simulink model "Model"  (R2023b)
settings: Solver=ode4  StartTime=0.0  StopTime=100  FixedStep=0.01  RelTol=1e-3
values from neighbouring files (symbols this model uses):
  D = sqrt(px*px + py*py)    [test2.m]
undefined symbols (not defined in the file or in its folder): X, Y, Z
libraries: nesl_utility x41, sm_lib x34, simulink_extras x10, sharedtransform x1
(part 2 of 2)

== matlab function Model/MATLAB Function1 ==
  data: theta input; J output
function J = jacobian_3link(theta)
    L0 = 0.04494;
    L1 = 0.08979;
    L2 = 0.1665;
    L3a = 0.02945;
    L3b = 0.1232;

    t0 = theta(1);
    t1 = theta(2);
    t2 = theta(3);
    t01 = t0 + t1;
    t012 = t01 + t2;

    Rp = @(theta) [-sin(theta); cos(theta)]; 

    J1 =  L0 * Rp(t0 + pi/2) ...
         +L1 * Rp(t0) ...
         +L2 * Rp(t01) ...
         +L3a * Rp(t012 + pi/2) ...
         +L3b * Rp(t012);

    J2 =  L2 * Rp(t01) ...
         +L3a * Rp(t012 + pi/2) ...
         +L3b * Rp(t012);

    J3 =  L3a * Rp(t012 + pi/2) ...
         +L3b * Rp(t012);

    J = [J1, J2, J3];
end

== matlab function Model/MATLAB Function ==
  data: theta input; pos output
function pos = fk_3link_explicit(theta)
    L0 = 0.04494;
    L1 = 0.08979;
    L2 = 0.1665;
    L3a = 0.02945;
    L3b = 0.1232;

    t0 = theta(1);
    t1 = theta(2);
    t2 = theta(3);
    t01 = t0 + t1;
    t012 = t01 + t2;

    R = @(theta) [cos(theta); sin(theta)];

    P0 = [0; 0];
    P1 = P0 + L0 * R(t0 + pi/2);
    P2 = P1 + L1 * R(t0);
    P3 = P2 + L2 * R(t01);
    P4 = P3 + L3a * R(t012 + pi/2);
    pos = P4 + L3b * R(t012);  % EE 위치
end

== matlab function Model/MATLAB Function2 ==
  data: theta input; thetad output
function thetad = ik_(theta)

t_pos = [0.2 0.2]';

pos_now = fk_3link_explicit(theta);

x = [pos_now(1), pos_now(2)]';

% x_des = 5*(t_pos - x);
x_des = [0 -0.02]';

J = jacobian_3link(theta);

Z = 1*[1 0 0]';

thetad  = pinv(J)*x_des + (eye(3,3) - pinv(J)*J)*Z;


end

function pos = fk_3link_explicit(theta)
    L0 = 0.04494;
    L1 = 0.08979;
    L2 = 0.1665;
    L3a = 0.02945;
    L3b = 0.1232;

    t0 = theta(1);
    t1 = theta(2);
    t2 = theta(3);
    t01 = t0 + t1;
    t012 = t01 + t2;

    R = @(theta) [cos(theta); sin(theta)];

    P0 = [0; 0];
    P1 = P0 + L0 * R(t0 + pi/2);
    P2 = P1 + L1 * R(t0);
    P3 = P2 + L2 * R(t01);
    P4 = P3 + L3a * R(t012 + pi/2);
    pos = P4 + L3b * R(t012);  % EE 위치
end

function J = jacobian_3link(theta)
    L0 = 0.04494;
    L1 = 0.08979;
    L2 = 0.1665;
    L3a = 0.02945;
    L3b = 0.1232;

    t0 = theta(1);
    t1 = theta(2);
    t2 = theta(3);
    t01 = t0 + t1;
    t012 = t01 + t2;

    Rp = @(theta) [-sin(theta); cos(theta)];  % 기존 부호 반전

    J1 =  L0 * Rp(t0 + pi/2) ...
         +L1 * Rp(t0) ...
         +L2 * Rp(t01) ...
         +L3a * Rp(t012 + pi/2) ...
         +L3b * Rp(t012);

    J2 =  L2 * Rp(t01) ...
         +L3a * Rp(t012 + pi/2) ...
         +L3b * Rp(t012);

    J3 =  L3a * Rp(t012 + pi/2) ...
         +L3b * Rp(t012);

    J = [J1, J2, J3];
end

== matlab function Model/MATLAB Function3 ==
  data: t input; res output
function res = ik_(t)

open_bd = [90 115 -25]';
open_bd_next1 = [0 0 0]';
open_bd_next  = [0 0 0]';
if t <= 10
    res = open_bd - [0; 10*(t/10); -25*(t/10)];
elseif ((t>10) && (t<20))
    open_bd = [90 105 0]';
    res = open_bd - [0; 15*((t-10)/10); 0*((t-10)/10)];
else
    open_bd = [90 90 0]';

    res = open_bd - [180*((t-20)/10); 90*((t-20)/10); 25*((t-20)/10)];

end





end

== matlab function Model/MATLAB Function5 ==
  data: cmd input; t_cmd output; cmd_d input; t_mea input; vd_mea input; v_mea input; p_mea input; mode input; tc_gain input; vc_gain input; pc_gain input; dt input
function t_cmd = motor_control(cmd,cmd_d, t_mea, vd_mea, v_mea, p_mea, mode, tc_gain, vc_gain, pc_gain, dt)

% persistent I_save
% persistent first_flg
% persistent mode_save
% 
% if isempty(first_flg)
%     first_flg = 1;
%     I_save = 0;
%     mode_save = 0;
% end
% 
% if mode_save ~= mode
%     mode_save = mode;
%     I_save = 0;
% end


if(mode == 1)%torque control
    % cmd : torque command [Nm]
    kp = tc_gain(1);
    ki = tc_gain(2);
    err = cmd - t_mea;

    % t_cmd = (kp*err) + (ki*I_save);
    t_cmd = (kp*err);
    % I_save = I_save + err*dt;

elseif(mode == 2) %velocity control
    % cmd : velocity command [rad/s]
    kp = vc_gain(1);
    ki = vc_gain(2);
    kd = vc_gain(3);

    err = cmd - v_mea;
    errd = cmd_d - vd_mea;
    % t_cmd = (kp*err) + (kd*errd);
    t_cmd = (kp*err) + (kd*errd);
elseif(mode == 3) %position control : position command [rad]
    kp = pc_gain(1);
    ki = pc_gain(2);
    kd = pc_gain(3);

    err = cmd - p_mea;
    errd = cmd_d - v_mea;
    % t_cmd = (kp*err) + (kd*errd) + (ki*I_save);
    t_cmd = (kp*err) + (kd*errd);
    % I_save = I_save + err*dt;
else%torque control
    t_cmd = 0;
end



end

== matlab function Model/MATLAB Function6 ==
  data: cmd input; t_cmd output; cmd_d input; t_mea input; vd_mea input; v_mea input; p_mea input; mode input; tc_gain input; vc_gain input; pc_gain input; dt input
function t_cmd = motor_control(cmd,cmd_d, t_mea, vd_mea, v_mea, p_mea, mode, tc_gain, vc_gain, pc_gain, dt)

% persistent I_save
% persistent first_flg
% persistent mode_save

% if isempty(first_flg)
%     first_flg = 1;
%     I_save = 0;
%     mode_save = 0;
% end
% 
% if mode_save ~= mode
%     mode_save = mode;
%     I_save = 0;
% end


if(mode == 1)%torque control
    % cmd : torque command [Nm]
    kp = tc_gain(1);
    ki = tc_gain(2);
    err = cmd - t_mea;

    % t_cmd = (kp*err) + (ki*I_save);
    t_cmd = (kp*err);
    % I_save = I_save + err*dt;

elseif(mode == 2) %velocity control
    % cmd : velocity command [rad/s]
    kp = vc_gain(1);
    ki = vc_gain(2);
    kd = vc_gain(3);

    err = cmd - v_mea;
    errd = cmd_d - vd_mea;
    % t_cmd = (kp*err) + (kd*errd);
    t_cmd = (kp*err) + (kd*errd);
elseif(mode == 3) %position control : position command [rad]
    kp = pc_gain(1);
    ki = pc_gain(2);
    kd = pc_gain(3);

    err = cmd - p_mea;
    errd = cmd_d - v_mea;
    % t_cmd = (kp*err) + (kd*errd) + (ki*I_save);
    t_cmd = (kp*err) + (kd*errd);
    % I_save = I_save + err*dt;
else%torque control
    t_cmd = 0;
end



end

== matlab function Model/MATLAB Function4 ==
  data: cmd input; t_cmd output; cmd_d input; t_mea input; vd_mea input; v_mea input; p_mea input; mode input; tc_gain input; vc_gain input; pc_gain input; dt input
function t_cmd = motor_control(cmd,cmd_d, t_mea, vd_mea, v_mea, p_mea, mode, tc_gain, vc_gain, pc_gain, dt)

% persistent I_save
% persistent first_flg
% persistent mode_save
% 
% if isempty(first_flg)
%     first_flg = 1;
%     I_save = 0;
%     mode_save = 0;
% end
% 
% if mode_save ~= mode
%     mode_save = mode;
%     I_save = 0;
% end


if(mode == 1)%torque control
    % cmd : torque command [Nm]
    kp = tc_gain(1);
    ki = tc_gain(2);
    err = cmd - t_mea;

    % t_cmd = (kp*err) + (ki*I_save);
    t_cmd = (kp*err);
    % I_save = I_save + err*dt;

elseif(mode == 2) %velocity control
    % cmd : velocity command [rad/s]
    kp = vc_gain(1);
    ki = vc_gain(2);
    kd = vc_gain(3);

    err = cmd - v_mea;
    errd = cmd_d - vd_mea;
    % t_cmd = (kp*err) + (kd*errd);
    t_cmd = (kp*err) + (kd*errd);
elseif(mode == 3) %position control : position command [rad]
    kp = pc_gain(1);
    ki = pc_gain(2);
    kd = pc_gain(3);

    err = cmd - p_mea;
    errd = cmd_d - v_mea;
    % t_cmd = (kp*err) + (kd*errd) + (ki*I_save);
    t_cmd = (kp*err) + (kd*errd);
    % I_save = I_save + err*dt;
else%torque control
    t_cmd = 0;
end



end
